simulink model "quarter_car"  (R2025a)
settings: Solver=ode4  StartTime=0.0  StopTime=t(end)  FixedStep=dt  RelTol=1e-3
values from neighbouring files (symbols this model uses):
  dt = 0.005    [Final_CSV.m]    (also in Single_Profile_Check.m = t(2) - t(1))
  ks = 16000    [Final_CSV.m]    (also in Single_Profile_Check.m)
  kt = 190000    [Final_CSV.m]    (also in Single_Profile_Check.m)
  ms = 290    [Final_CSV.m]    (also in Single_Profile_Check.m)
  mu = 59    [Final_CSV.m]    (also in Single_Profile_Check.m)
libraries: simulink x2
settings Model: Creator=Dell  LastModifiedBy=Dell
settings RTWCC: RTWVerbose=off

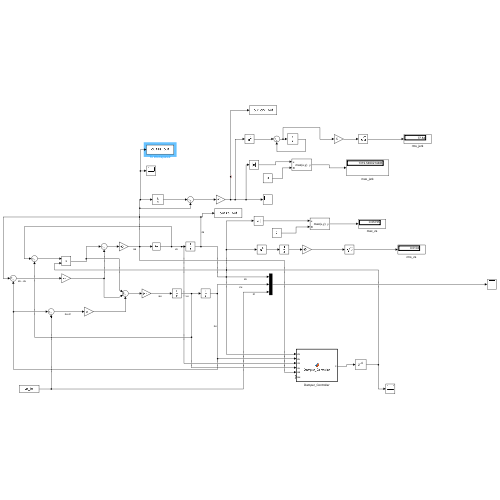
[thumbnail: Simulink's stored preview of the top-level diagram]
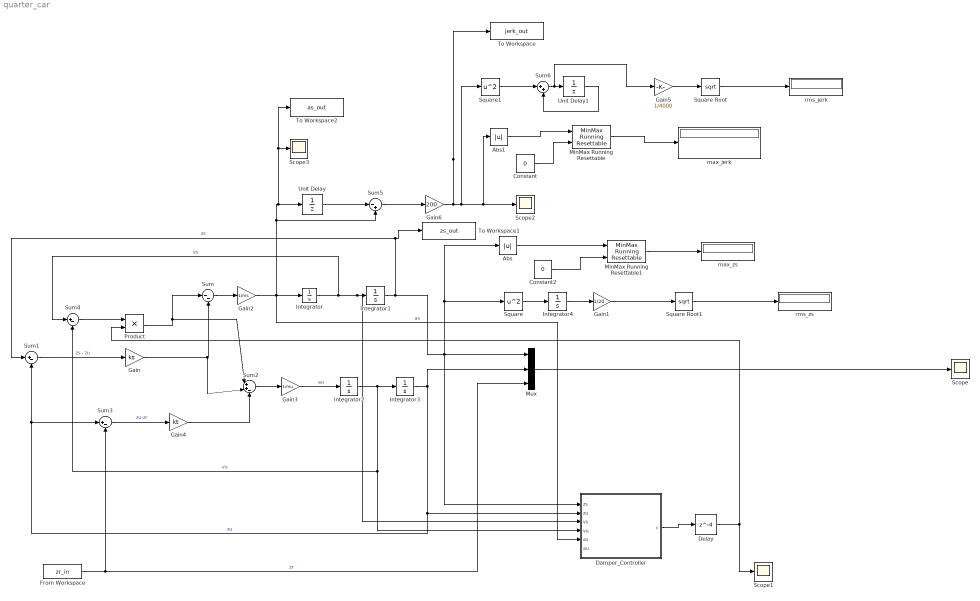
== system quarter_car ==
  Abs : Abs  SaturateOnIntegerOverflow=off
  Abs1 : Abs  SaturateOnIntegerOverflow=off
  Constant : Constant  Value=0
  Constant2 : Constant  Value=0
  Damper_Controller : MATLAB Function  TreatAsAtomicUnit=on
  Delay : Delay  DelayLength=4  InitialCondition=800  SampleTime=dt
  From Workspace : FromWorkspace  VariableName=zr_in
  Gain : Gain  Gain=ks
  Gain1 : Gain  Gain=1/20
  Gain2 : Gain  Gain=1/ms
  Gain3 : Gain  Gain=1/mu
  Gain4 : Gain  Gain=kt
  Gain5 : Gain  Gain=1/4000
  Gain6 : Gain  Gain=200
  Integrator{,1..4} (5 alike) : Integrator
  MinMax Running Resettable : simulink/Math Operations/MinMax Running Resettable  Function=max  vinit=0.0
  MinMax Running Resettable1 : simulink/Math Operations/MinMax Running Resettable  Function=max  vinit=0.0
  Mux : Mux  Inputs=3
  Product : Product
  Scope{,1..3} (4 alike) : Scope
      Scope settings: ActiveDisplayYMinimum=-0.02645297077792283  ActiveDisplayYMaximum=0.10578606107746077
      Scope1 settings: ActiveDisplayYMinimum=682.86784201759065  ActiveDisplayYMaximum=3715.2314184904294
      Scope2 settings: ActiveDisplayYMinimum=-183.89487386384451  ActiveDisplayYMaximum=-182.4909790536295  DataLoggingVariableName=ScopeData2
      Scope3 settings: ActiveDisplayYMinimum=-24.800500324385872  ActiveDisplayYMaximum=24.220090230065455  DataLoggingVariableName=ScopeData3
  Square : Math  Operator=square
  Square Root : Sqrt
  Square Root1 : Sqrt
  Square1 : Math  Operator=square
  Sum : Sum  Inputs=|--
  Sum1 : Sum  Inputs=|+-
  Sum2 : Sum  Inputs=|++-
  Sum3 : Sum  Inputs=|+-
  Sum4 : Sum  Inputs=|+-
  Sum5 : Sum  Inputs=|-+
  Sum6 : Sum  Inputs=|++
  To Workspace : ToWorkspace  VariableName=jerk_out  SampleTime=-1
  To Workspace1 : ToWorkspace  VariableName=zs_out  SampleTime=-1
  To Workspace2 : ToWorkspace  VariableName=as_out  SampleTime=-1
  Unit Delay : UnitDelay  SampleTime=dt  HasFrameUpgradeWarning=on
  Unit Delay1 : UnitDelay  SampleTime=dt  HasFrameUpgradeWarning=on
  max_jerk : Display
      settings: Decimation=8
  max_zs : Display
  rms_jerk : Display
  rms_zs : Display
  wires:
  Sum1/1 -> Gain/1  "zs - zu"
  Sum4/1 -> Product/1
  Product/1 -> Sum2/1, Sum/1
  Gain/1 -> Sum2/2, Sum/2
  Sum/1 -> Gain2/1
  Gain2/1 -> Sum5/2, Unit Delay/1, To Workspace2/1, Scope3/1, Damper_Controller/5(as), Integrator/1  "as"
  Sum2/1 -> Gain3/1
  Gain3/1 -> Integrator2/1  "au"
  Gain4/1 -> Sum2/3
  Integrator/1 -> Damper_Controller/3(vs), Integrator1/1, Sum4/1  "vs"
  Integrator2/1 -> Damper_Controller/4(vu), Sum4/2, Integrator3/1  "vu"
  Integrator3/1 -> Mux/2, Damper_Controller/2(zu), Sum3/1, Sum1/2  "zu"
  Integrator1/1 -> Square/1, Abs/1, Damper_Controller/1(zs), Mux/1, To Workspace1/1, Sum1/1  "zs"
  Sum3/1 -> Gain4/1  "zu-zr"
  From Workspace/1 -> Mux/3, Sum3/2  "zr"
  Mux/1 -> Scope/1
  Damper_Controller/1(c) -> Delay/1
  Delay/1 -> Scope1/1, Product/2
  Gain6/1 -> To Workspace/1, Square1/1, Abs1/1, Scope2/1
  Abs1/1 -> MinMax Running Resettable/1
  Abs/1 -> MinMax Running Resettable1/1
  Square/1 -> Integrator4/1
  Integrator4/1 -> Gain1/1
  Gain1/1 -> Square Root1/1
  Unit Delay/1 -> Sum5/1
  Sum5/1 -> Gain6/1
  Square1/1 -> Sum6/1
  Gain5/1 -> Square Root/1
  Square Root1/1 -> rms_zs/1
  MinMax Running Resettable/1 -> max_jerk/1
  Square Root/1 -> rms_jerk/1
  MinMax Running Resettable1/1 -> max_zs/1
  Constant/1 -> MinMax Running Resettable/2
  Constant2/1 -> MinMax Running Resettable1/2
  Sum6/1 -> Gain5/1, Unit Delay1/1
  Unit Delay1/1 -> Sum6/2

== matlab function quarter_car/Damper_Controller ==
  settings: updateMethod=DISCRETE  sampleTime=0.02
  data: zs input; c output; zu input; vs input; vu input; as input; au input
function c = Damper_Controller(zs, zu, vs, vu, as, au)

c_min = 800;
c_mid = 1500;
c_max = 3200;

a_th = 1.5;
z_th = 0.02;

T_hold = 0.1;
Ts = 0.02;

persistent impact_timer
if isempty(impact_timer)
    impact_timer = 0;
end

z_rel = zs - zu;
v_rel = vs - vu;

impact = (abs(as) > a_th) || (abs(z_rel) > z_th);

if impact
    impact_timer = T_hold;
else
    impact_timer = max(impact_timer - 1.5*Ts, 0);
end

compression = (z_rel < 0) && (v_rel > 0);
rebound     = (z_rel > 0) && (v_rel > 0);

body_ok  = (as * v_rel) > 0;
wheel_ok = (au * v_rel) < 0;

if impact_timer > 0
    c = c_max;

elseif rebound
    c = 0.8 * c_max;

elseif body_ok && wheel_ok
    c = c_mid;

else
    c = c_min;
end

end
